simulink model "VVI"  (R2023a)
settings: Solver=FixedStepAuto  StartTime=0.0  StopTime=10.0  FixedStep=0.001  RelTol=1e-3  EnableMultiTasking=on
settings Model: ExtModeTrigDuration=5  Creator=tstic  LastModifiedBy=tstic
settings OptimizationCC: EnhancedBackFolding=on  PassReuseOutputArgsAs=Individual arguments  ZeroExternalMemoryAtStartup=off  ZeroInternalMemoryAtStartup=off  MaxStackSize=64  OptimizeBlockOrder=speed  DifferentSizesBufferReuse=on  OptimizationCustomize=off  EfficientTunableParamExpr=on
settings DebuggingCC: ParameterTunabilityLossMsg=error
settings HardwareCC: ProdBitPerPointer=32  ProdBitPerSizeT=32  ProdBitPerPtrDiffT=32  ProdLargestAtomicInteger=Long  ProdLargestAtomicFloat=Double  ProdWordSize=32  ProdHWDeviceType=ARM Compatible->ARM Cortex
settings SFSimCC: MATLABDynamicMemAlloc=off
settings RTWCC: Description=Embedded Coder  SystemTargetFile=ert.tlc  HardwareBoard=NXP FRDM-K64F  TLCOptions="-aInlineSetEventsForThisBaseRateFcn=TLC_FALSE -aSuppressMultiTaskScheduler=TLC_FALSE  -aRateBasedStepFcn=0"  TemplateMakefile=ert_default_tmf  Toolchain=GNU Tools for ARM Embedded Processors
settings CodeAppCC: ForceParamTrailComments=on  IgnoreCustomStorageClasses=off  OperatorAnnotations=on  SimulinkDataObjDesc=on  SFDataObjDesc=on  InsertBlockDesc=on
settings ERTTargetCC: ExtModeTransport=4  ExtModeMexFile=sendToCommService

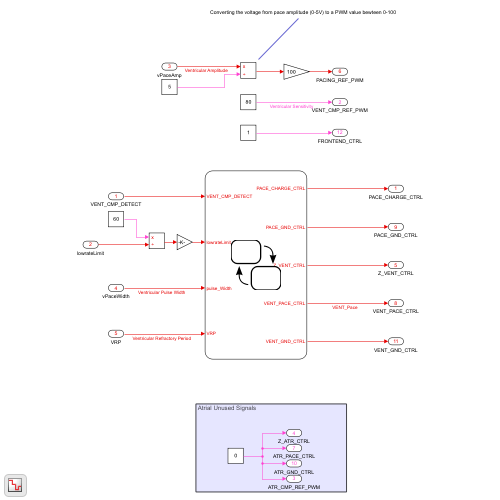
[thumbnail: Simulink's stored preview of the top-level diagram]
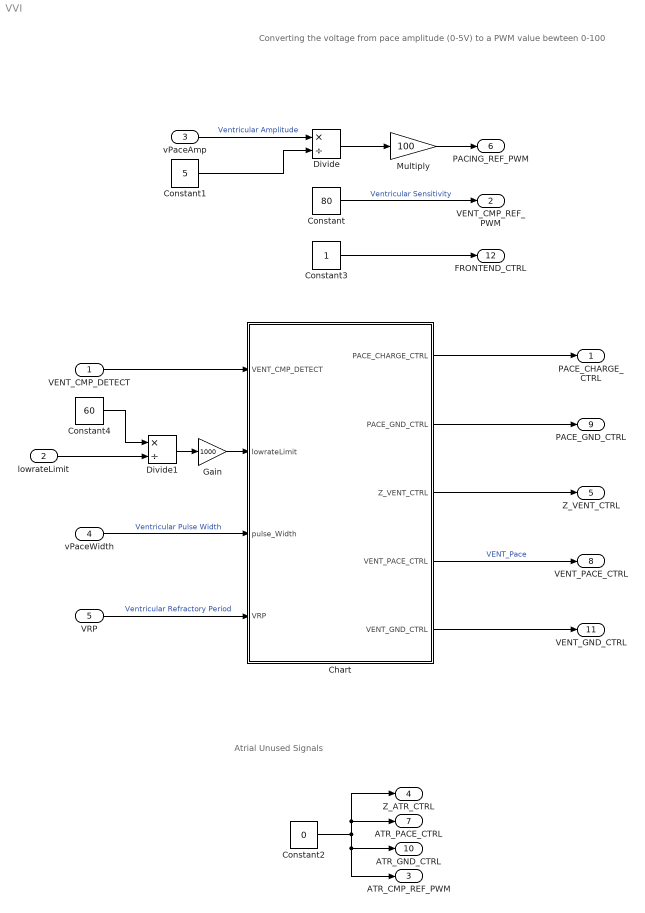
== system VVI ==
  note: Converting the voltage from pace amplitude (0-5V) to a PWM value bewteen 0-100
  note: Atrial Unused Signals
  VENT_CMP_DETECT : Inport  OutDataTypeStr=boolean
  lowrateLimit : Inport  Port=2  OutMin=[30]  OutMax=[175]
  vPaceAmp : Inport  Port=3
  vPaceWidth : Inport  Port=4
  VRP : Inport  Port=5
  Chart : Stateflow chart  TreatAsAtomicUnit=on
  Constant : Constant  Value=80
  Constant1 : Constant  Value=5
  Constant2 : Constant  Value=0
  Constant3 : Constant  OutDataTypeStr=Inherit: Inherit via back propagation
  Constant4 : Constant  Value=60
  Divide : Product  Inputs=*/
  Divide1 : Product  Inputs=*/
  Gain : Gain  Gain=1000
  Multiply : Gain  Gain=100
  PACE_CHARGE_CTRL : Outport
  VENT_CMP_REF_PWM : Outport  Port=2
  ATR_CMP_REF_PWM : Outport  Port=3
  Z_ATR_CTRL : Outport  Port=4
  Z_VENT_CTRL : Outport  Port=5
  PACING_REF_PWM : Outport  Port=6
  ATR_PACE_CTRL : Outport  Port=7
  VENT_PACE_CTRL : Outport  Port=8
  PACE_GND_CTRL : Outport  Port=9
  ATR_GND_CTRL : Outport  Port=10
  VENT_GND_CTRL : Outport  Port=11
  FRONTEND_CTRL : Outport  Port=12
  wires:
  Constant2/1 -> ATR_CMP_REF_PWM/1, ATR_GND_CTRL/1, Z_ATR_CTRL/1, ATR_PACE_CTRL/1
  VENT_CMP_DETECT/1 -> Chart/1(VENT_CMP_DETECT)
  Chart/1(PACE_CHARGE_CTRL) -> PACE_CHARGE_CTRL/1
  Chart/2(PACE_GND_CTRL) -> PACE_GND_CTRL/1
  Chart/3(Z_VENT_CTRL) -> Z_VENT_CTRL/1
  Chart/4(VENT_PACE_CTRL) -> VENT_PACE_CTRL/1  "VENT_Pace"
  Chart/5(VENT_GND_CTRL) -> VENT_GND_CTRL/1
  Constant/1 -> VENT_CMP_REF_PWM/1  "Ventricular Sensitivity"
  Constant3/1 -> FRONTEND_CTRL/1
  vPaceWidth/1 -> Chart/3(pulse_Width)  "Ventricular Pulse Width"
  Multiply/1 -> PACING_REF_PWM/1
  Divide/1 -> Multiply/1
  Constant1/1 -> Divide/2
  vPaceAmp/1 -> Divide/1  "Ventricular Amplitude"
  lowrateLimit/1 -> Divide1/2
  VRP/1 -> Chart/4(VRP)  "Ventricular Refractory Period"
  Divide1/1 -> Gain/1
  Constant4/1 -> Divide1/1
  Gain/1 -> Chart/2(lowrateLimit)

== stateflow chart VVI/Chart ==
  note: If there hasn't been a ventrical pace within the low rate interval then pace the ventricle
  state Charging% and discharging Blocking Cap
    entry:
    PACE_GND_CTRL = true;
    VENT_GND_CTRL = true;
    Z_VENT_CTRL = false;
    during:
    PACE_CHARGE_CTRL = true;
  state Pace
    entry:
    PACE_CHARGE_CTRL = false;
    VENT_GND_CTRL = false;
    PACE_GND_CTRL = true;
    Z_VENT_CTRL = false;
    VENT_PACE_CTRL = true;
  note: Pace the ventricle for the duration of the pulse width
  note: prevent trigger/inhibition whenever
      | a ventricle pace is detected for the
      | duration of the VRP
  (default) -> Charging% and discharging Blocking Cap
  Charging% and discharging Blocking Cap -> Pace [order 1] : [duration(VENT_CMP_DETECT == false,msec) > lowrateLimit]
  Pace -> Charging% and discharging Blocking Cap : after(pulse_Width,msec){VENT_PACE_CTRL = false;}
  Charging% and discharging Blocking Cap -> (junction 40) [order 2] : [VENT_CMP_DETECT]
  (junction 40) -> Charging% and discharging Blocking Cap : after(VRP,msec)
  data: VENT_CMP_DETECT input; lowrateLimit input; PACE_CHARGE_CTRL output; PACE_GND_CTRL output; Z_VENT_CTRL output; VENT_PACE_CTRL output; VENT_GND_CTRL output; pulse_Width input; VRP input
